simulink model "IEEE9_case"  (R2024b)
settings: Solver=FixedStepAuto  StartTime=0  StopTime=5  FixedStep=1e-7  RelTol=1e-3
values from neighbouring files (symbols this model uses):
  SG_D_1_D = 0.01056    [IEEE9_case_parameters.m]    (also in case1_parameters.m; case2_parameters.m; case3_parameters.m; case4_parameters.m)
  SG_D_1_EnableSaturation = 0    [IEEE9_case_parameters.m]    (also in case1_parameters.m; case2_parameters.m; case3_parameters.m; case4_parameters.m)
  SG_D_1_f0 = 60    [IEEE9_case_parameters.m]    (also in case1_parameters.m; case2_parameters.m; case3_parameters.m; case4_parameters.m)
  SG_D_1_H = 7.5    [IEEE9_case_parameters.m]    (also in case1_parameters.m; case2_parameters.m; case3_parameters.m; case4_parameters.m)
  SG_D_1_K_A = 20    [IEEE9_case_parameters.m]    (also in case1_parameters.m; case2_parameters.m; case3_parameters.m; case4_parameters.m)
  SG_D_1_K_E = 1.000000e+1    (= 10)    [IEEE9_case_parameters.m]    (also in case1_parameters.m; case2_parameters.m; case3_parameters.m; case4_parameters.m)
  SG_D_1_K_F = 2.363    [IEEE9_case_parameters.m]    (also in case1_parameters.m; case2_parameters.m; case3_parameters.m; case4_parameters.m)
  SG_D_1_K_s = 0.5    [IEEE9_case_parameters.m]    (also in case1_parameters.m = 5; case2_parameters.m = 5; case3_parameters.m = 5; case4_parameters.m = 5)
  SG_D_1_R_a = 0.001088    [IEEE9_case_parameters.m]    (also in case1_parameters.m; case2_parameters.m; case3_parameters.m; case4_parameters.m)
  SG_D_1_S_A = 1    [IEEE9_case_parameters.m]    (also in case1_parameters.m; case2_parameters.m; case3_parameters.m; case4_parameters.m)
  SG_D_1_S_B = 0.103    [IEEE9_case_parameters.m]    (also in case1_parameters.m; case2_parameters.m; case3_parameters.m; case4_parameters.m)
  SG_D_1_S_N = 10.659857    [IEEE9_case_parameters.m]    (also in case1_parameters.m; case2_parameters.m; case3_parameters.m; case4_parameters.m)
  SG_D_1_SpeedPara = 200    [IEEE9_case_parameters.m]    (also in case1_parameters.m; case2_parameters.m; case3_parameters.m; case4_parameters.m)
  SG_D_1_T_0 = 0.720173    [IEEE9_case_parameters.m]    (also in case1_parameters.m = 0.755522; case2_parameters.m = 0.808931; case3_parameters.m = 0.869402; case4_parameters.m = 0.729316)
  SG_D_1_T_1 = 0.3    [IEEE9_case_parameters.m]    (also in case1_parameters.m; case2_parameters.m; case3_parameters.m; case4_parameters.m)
  SG_D_1_T_2 = 0.05    [IEEE9_case_parameters.m]    (also in case1_parameters.m; case2_parameters.m; case3_parameters.m; case4_parameters.m)
  SG_D_1_T_3 = 0.02    [IEEE9_case_parameters.m]    (also in case1_parameters.m; case2_parameters.m; case3_parameters.m; case4_parameters.m)
  SG_D_1_T_4 = 0.005    [IEEE9_case_parameters.m]    (also in case1_parameters.m; case2_parameters.m; case3_parameters.m; case4_parameters.m)
  SG_D_1_T_A = 0.02    [IEEE9_case_parameters.m]    (also in case1_parameters.m; case2_parameters.m; case3_parameters.m; case4_parameters.m)
  SG_D_1_T_dd = 8.000000e+0    (= 8)    [IEEE9_case_parameters.m]    (also in case1_parameters.m; case2_parameters.m; case3_parameters.m; case4_parameters.m)
  SG_D_1_T_ddd = 0.04    [IEEE9_case_parameters.m]    (also in case1_parameters.m; case2_parameters.m; case3_parameters.m; case4_parameters.m)
  SG_D_1_T_E = 0.314    [IEEE9_case_parameters.m]    (also in case1_parameters.m; case2_parameters.m; case3_parameters.m; case4_parameters.m)
  SG_D_1_T_F = 0.35    [IEEE9_case_parameters.m]    (also in case1_parameters.m; case2_parameters.m; case3_parameters.m; case4_parameters.m)
  SG_D_1_T_qd = 0.8    [IEEE9_case_parameters.m]    (also in case1_parameters.m; case2_parameters.m; case3_parameters.m; case4_parameters.m)
  SG_D_1_T_qdd = 0.02    [IEEE9_case_parameters.m]    (also in case1_parameters.m; case2_parameters.m; case3_parameters.m; case4_parameters.m)
  SG_D_1_T_speed = 0.1    [IEEE9_case_parameters.m]    (also in case1_parameters.m = 200; case2_parameters.m = 200; case3_parameters.m = 200; case4_parameters.m = 200)
  SG_D_1_T_w = 0.5    [IEEE9_case_parameters.m]    (also in case1_parameters.m; case2_parameters.m; case3_parameters.m; case4_parameters.m)
  SG_D_1_V_ref = 1.990276    [IEEE9_case_parameters.m]    (also in case1_parameters.m = 2.042296; case2_parameters.m = 2.051388; case3_parameters.m = 2.089584; case4_parameters.m = 2.01845)
  SG_D_1_w_ref = 376.991118    [IEEE9_case_parameters.m]    (also in case1_parameters.m; case2_parameters.m; case3_parameters.m; case4_parameters.m)
  SG_D_1_wb = 6.000000e+1    (= 60)    [IEEE9_case_parameters.m]    (also in case1_parameters.m; case2_parameters.m; case3_parameters.m; case4_parameters.m)
  SG_D_1_x_d = 1.9    [IEEE9_case_parameters.m]    (also in case1_parameters.m; case2_parameters.m; case3_parameters.m; case4_parameters.m)
  SG_D_1_x_dd = 0.302    [IEEE9_case_parameters.m]    (also in case1_parameters.m; case2_parameters.m; case3_parameters.m; case4_parameters.m)
  SG_D_1_x_ddd = 0.204    [IEEE9_case_parameters.m]    (also in case1_parameters.m; case2_parameters.m; case3_parameters.m; case4_parameters.m)
  SG_D_1_x_l = 0.05    [IEEE9_case_parameters.m]    (also in case1_parameters.m; case2_parameters.m; case3_parameters.m; case4_parameters.m)
  SG_D_1_x_q = 1.3    [IEEE9_case_parameters.m]    (also in case1_parameters.m; case2_parameters.m; case3_parameters.m; case4_parameters.m)
  SG_D_1_x_qd = 0.5    [IEEE9_case_parameters.m]    (also in case1_parameters.m; case2_parameters.m; case3_parameters.m; case4_parameters.m)
  SG_D_1_x_qdd = 0.3    [IEEE9_case_parameters.m]    (also in case1_parameters.m; case2_parameters.m; case3_parameters.m; case4_parameters.m)
  SG_D_2_D = 0.02    [IEEE9_case_parameters.m]    (also in case1_parameters.m; case2_parameters.m; case3_parameters.m; case4_parameters.m)
  SG_D_2_EnableSaturation = 0    [IEEE9_case_parameters.m]    (also in case1_parameters.m; case2_parameters.m; case3_parameters.m; case4_parameters.m)
  SG_D_2_f0 = 60    [IEEE9_case_parameters.m]    (also in case1_parameters.m; case2_parameters.m; case3_parameters.m; case4_parameters.m)
  SG_D_2_H = 8.000000e+0    (= 8)    [IEEE9_case_parameters.m]    (also in case1_parameters.m; case2_parameters.m; case3_parameters.m; case4_parameters.m)
  SG_D_2_K_A = 20    [IEEE9_case_parameters.m]    (also in case1_parameters.m; case2_parameters.m; case3_parameters.m; case4_parameters.m)
  SG_D_2_K_E = 1.000000e+1    (= 10)    [IEEE9_case_parameters.m]    (also in case1_parameters.m; case2_parameters.m; case3_parameters.m; case4_parameters.m)
  SG_D_2_K_F = 2.363    [IEEE9_case_parameters.m]    (also in case1_parameters.m; case2_parameters.m; case3_parameters.m; case4_parameters.m)
  SG_D_2_K_s = 0.5    [IEEE9_case_parameters.m]    (also in case1_parameters.m = 4; case2_parameters.m = 4; case3_parameters.m = 4; case4_parameters.m = 4)
  SG_D_2_R_a = 0.001088    [IEEE9_case_parameters.m]    (also in case1_parameters.m; case2_parameters.m; case3_parameters.m; case4_parameters.m)
  SG_D_2_S_A = 1    [IEEE9_case_parameters.m]    (also in case1_parameters.m; case2_parameters.m; case3_parameters.m; case4_parameters.m)
  SG_D_2_S_B = 0.103    [IEEE9_case_parameters.m]    (also in case1_parameters.m; case2_parameters.m; case3_parameters.m; case4_parameters.m)
  SG_D_2_S_N = 10.659857    [IEEE9_case_parameters.m]    (also in case1_parameters.m; case2_parameters.m; case3_parameters.m; case4_parameters.m)
  SG_D_2_SpeedPara = 200    [IEEE9_case_parameters.m]    (also in case1_parameters.m; case2_parameters.m; case3_parameters.m; case4_parameters.m)
  SG_D_2_T_0 = 1.632913    [IEEE9_case_parameters.m]    (also in case1_parameters.m = 1.632925; case2_parameters.m = 1.632915; case3_parameters.m = 1.632914; case4_parameters.m = 1.632927)
  SG_D_2_T_1 = 0.2    [IEEE9_case_parameters.m]    (also in case1_parameters.m; case2_parameters.m; case3_parameters.m; case4_parameters.m)
  SG_D_2_T_2 = 0.05    [IEEE9_case_parameters.m]    (also in case1_parameters.m; case2_parameters.m; case3_parameters.m; case4_parameters.m)
  SG_D_2_T_3 = 0.02    [IEEE9_case_parameters.m]    (also in case1_parameters.m; case2_parameters.m; case3_parameters.m; case4_parameters.m)
  SG_D_2_T_4 = 0.005    [IEEE9_case_parameters.m]    (also in case1_parameters.m; case2_parameters.m; case3_parameters.m; case4_parameters.m)
  SG_D_2_T_A = 0.02    [IEEE9_case_parameters.m]    (also in case1_parameters.m; case2_parameters.m; case3_parameters.m; case4_parameters.m)
  SG_D_2_T_dd = 7.9    [IEEE9_case_parameters.m]    (also in case1_parameters.m; case2_parameters.m; case3_parameters.m; case4_parameters.m)
  SG_D_2_T_ddd = 0.04    [IEEE9_case_parameters.m]    (also in case1_parameters.m; case2_parameters.m; case3_parameters.m; case4_parameters.m)
  SG_D_2_T_E = 0.314    [IEEE9_case_parameters.m]    (also in case1_parameters.m; case2_parameters.m; case3_parameters.m; case4_parameters.m)
  SG_D_2_T_F = 0.35    [IEEE9_case_parameters.m]    (also in case1_parameters.m; case2_parameters.m; case3_parameters.m; case4_parameters.m)
  SG_D_2_T_qd = 0.8    [IEEE9_case_parameters.m]    (also in case1_parameters.m; case2_parameters.m; case3_parameters.m; case4_parameters.m)
  SG_D_2_T_qdd = 0.015    [IEEE9_case_parameters.m]    (also in case1_parameters.m; case2_parameters.m; case3_parameters.m; case4_parameters.m)
  SG_D_2_T_speed = 0.1    [IEEE9_case_parameters.m]    (also in case1_parameters.m = 150; case2_parameters.m = 150; case3_parameters.m = 150; case4_parameters.m = 150)
  SG_D_2_T_w = 0.35    [IEEE9_case_parameters.m]    (also in case1_parameters.m; case2_parameters.m; case3_parameters.m; case4_parameters.m)
  SG_D_2_V_ref = 2.58547    [IEEE9_case_parameters.m]    (also in case1_parameters.m = 2.597896; case2_parameters.m = 2.587136; case3_parameters.m = 2.586042; case4_parameters.m = 2.599679)
  SG_D_2_w_ref = 376.991118    [IEEE9_case_parameters.m]    (also in case1_parameters.m; case2_parameters.m; case3_parameters.m; case4_parameters.m)
  SG_D_2_wb = 6.000000e+1    (= 60)    [IEEE9_case_parameters.m]    (also in case1_parameters.m; case2_parameters.m; case3_parameters.m; case4_parameters.m)
  SG_D_2_x_d = 1.8    [IEEE9_case_parameters.m]    (also in case1_parameters.m; case2_parameters.m; case3_parameters.m; case4_parameters.m)
  SG_D_2_x_dd = 0.302    [IEEE9_case_parameters.m]    (also in case1_parameters.m; case2_parameters.m; case3_parameters.m; case4_parameters.m)
  SG_D_2_x_ddd = 0.204    [IEEE9_case_parameters.m]    (also in case1_parameters.m; case2_parameters.m; case3_parameters.m; case4_parameters.m)
  SG_D_2_x_l = 0.05    [IEEE9_case_parameters.m]    (also in case1_parameters.m; case2_parameters.m; case3_parameters.m; case4_parameters.m)
  SG_D_2_x_q = 1.25    [IEEE9_case_parameters.m]    (also in case1_parameters.m; case2_parameters.m; case3_parameters.m; case4_parameters.m)
  SG_D_2_x_qd = 0.5    [IEEE9_case_parameters.m]    (also in case1_parameters.m; case2_parameters.m; case3_parameters.m; case4_parameters.m)
  SG_D_2_x_qdd = 0.3    [IEEE9_case_parameters.m]    (also in case1_parameters.m; case2_parameters.m; case3_parameters.m; case4_parameters.m)
  SG_D_3_D = 0.02    [IEEE9_case_parameters.m]    (also in case1_parameters.m; case2_parameters.m; case3_parameters.m; case4_parameters.m)
  SG_D_3_EnableSaturation = 0    [IEEE9_case_parameters.m]    (also in case1_parameters.m; case2_parameters.m; case3_parameters.m; case4_parameters.m)
  SG_D_3_f0 = 60    [IEEE9_case_parameters.m]    (also in case1_parameters.m; case2_parameters.m; case3_parameters.m; case4_parameters.m)
  SG_D_3_H = 7.7    [IEEE9_case_parameters.m]    (also in case1_parameters.m; case2_parameters.m; case3_parameters.m; case4_parameters.m)
  SG_D_3_K_A = 20    [IEEE9_case_parameters.m]    (also in case1_parameters.m; case2_parameters.m; case3_parameters.m; case4_parameters.m)
  SG_D_3_K_E = 1.000000e+1    (= 10)    [IEEE9_case_parameters.m]    (also in case1_parameters.m; case2_parameters.m; case3_parameters.m; case4_parameters.m)
  SG_D_3_K_F = 2.363    [IEEE9_case_parameters.m]    (also in case1_parameters.m; case2_parameters.m; case3_parameters.m; case4_parameters.m)
  SG_D_3_K_s = 0.2    [IEEE9_case_parameters.m]    (also in case1_parameters.m = 2; case2_parameters.m = 2; case3_parameters.m = 2; case4_parameters.m = 2)
  SG_D_3_R_a = 0.001088    [IEEE9_case_parameters.m]    (also in case1_parameters.m; case2_parameters.m; case3_parameters.m; case4_parameters.m)
  SG_D_3_S_A = 1    [IEEE9_case_parameters.m]    (also in case1_parameters.m; case2_parameters.m; case3_parameters.m; case4_parameters.m)
  SG_D_3_S_B = 0.103    [IEEE9_case_parameters.m]    (also in case1_parameters.m; case2_parameters.m; case3_parameters.m; case4_parameters.m)
  SG_D_3_S_N = 10.659857    [IEEE9_case_parameters.m]    (also in case1_parameters.m; case2_parameters.m; case3_parameters.m; case4_parameters.m)
  SG_D_3_SpeedPara = 200    [IEEE9_case_parameters.m]    (also in case1_parameters.m; case2_parameters.m; case3_parameters.m; case4_parameters.m)
  SG_D_3_T_0 = 0.850788    [IEEE9_case_parameters.m]    (also in case1_parameters.m = 0.850786; case2_parameters.m = 0.850787; case3_parameters.m; case4_parameters.m = 0.850786)
  SG_D_3_T_1 = 0.2    [IEEE9_case_parameters.m]    (also in case1_parameters.m; case2_parameters.m; case3_parameters.m; case4_parameters.m)
  SG_D_3_T_2 = 0.05    [IEEE9_case_parameters.m]    (also in case1_parameters.m; case2_parameters.m; case3_parameters.m; case4_parameters.m)
  SG_D_3_T_3 = 0.02    [IEEE9_case_parameters.m]    (also in case1_parameters.m; case2_parameters.m; case3_parameters.m; case4_parameters.m)
  SG_D_3_T_4 = 0.005    [IEEE9_case_parameters.m]    (also in case1_parameters.m; case2_parameters.m; case3_parameters.m; case4_parameters.m)
  SG_D_3_T_A = 0.02    [IEEE9_case_parameters.m]    (also in case1_parameters.m; case2_parameters.m; case3_parameters.m; case4_parameters.m)
  SG_D_3_T_dd = 8.1    [IEEE9_case_parameters.m]    (also in case1_parameters.m; case2_parameters.m; case3_parameters.m; case4_parameters.m)
  SG_D_3_T_ddd = 0.04    [IEEE9_case_parameters.m]    (also in case1_parameters.m; case2_parameters.m; case3_parameters.m; case4_parameters.m)
  SG_D_3_T_E = 0.314    [IEEE9_case_parameters.m]    (also in case1_parameters.m; case2_parameters.m; case3_parameters.m; case4_parameters.m)
  SG_D_3_T_F = 0.35    [IEEE9_case_parameters.m]    (also in case1_parameters.m; case2_parameters.m; case3_parameters.m; case4_parameters.m)
  SG_D_3_T_qd = 0.8    [IEEE9_case_parameters.m]    (also in case1_parameters.m; case2_parameters.m; case3_parameters.m; case4_parameters.m)
  SG_D_3_T_qdd = 0.015    [IEEE9_case_parameters.m]    (also in case1_parameters.m; case2_parameters.m; case3_parameters.m; case4_parameters.m)
  SG_D_3_T_speed = 0.1    [IEEE9_case_parameters.m]    (also in case1_parameters.m = 180; case2_parameters.m = 180; case3_parameters.m = 180; case4_parameters.m = 180)
  SG_D_3_T_w = 0.4    [IEEE9_case_parameters.m]    (also in case1_parameters.m; case2_parameters.m; case3_parameters.m; case4_parameters.m)
  SG_D_3_V_ref = 1.892727    [IEEE9_case_parameters.m]    (also in case1_parameters.m = 1.906439; case2_parameters.m = 1.895535; case3_parameters.m = 1.892105; case4_parameters.m = 1.906598)
  SG_D_3_w_ref = 376.991118    [IEEE9_case_parameters.m]    (also in case1_parameters.m; case2_parameters.m; case3_parameters.m; case4_parameters.m)
  SG_D_3_wb = 6.000000e+1    (= 60)    [IEEE9_case_parameters.m]    (also in case1_parameters.m; case2_parameters.m; case3_parameters.m; case4_parameters.m)
  SG_D_3_x_d = 1.85    [IEEE9_case_parameters.m]    (also in case1_parameters.m; case2_parameters.m; case3_parameters.m; case4_parameters.m)
  SG_D_3_x_dd = 0.302    [IEEE9_case_parameters.m]    (also in case1_parameters.m; case2_parameters.m; case3_parameters.m; case4_parameters.m)
  SG_D_3_x_ddd = 0.204    [IEEE9_case_parameters.m]    (also in case1_parameters.m; case2_parameters.m; case3_parameters.m; case4_parameters.m)
  SG_D_3_x_l = 0.05    [IEEE9_case_parameters.m]    (also in case1_parameters.m; case2_parameters.m; case3_parameters.m; case4_parameters.m)
  SG_D_3_x_q = 1.2    [IEEE9_case_parameters.m]    (also in case1_parameters.m; case2_parameters.m; case3_parameters.m; case4_parameters.m)
  SG_D_3_x_qd = 0.5    [IEEE9_case_parameters.m]    (also in case1_parameters.m; case2_parameters.m; case3_parameters.m; case4_parameters.m)
  SG_D_3_x_qdd = 0.3    [IEEE9_case_parameters.m]    (also in case1_parameters.m; case2_parameters.m; case3_parameters.m; case4_parameters.m)
(part 1 of 12)
settings Model: SimulationMode=accelerator  Creator=Greg  LastModifiedBy=Greg
settings DataIOCC: ReturnWorkspaceOutputs=off

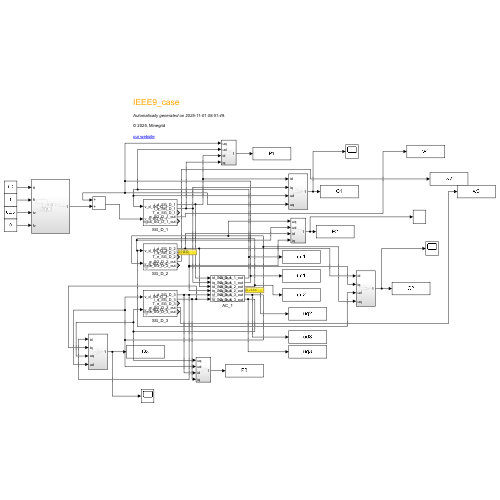
[thumbnail: Simulink's stored preview of the top-level diagram]
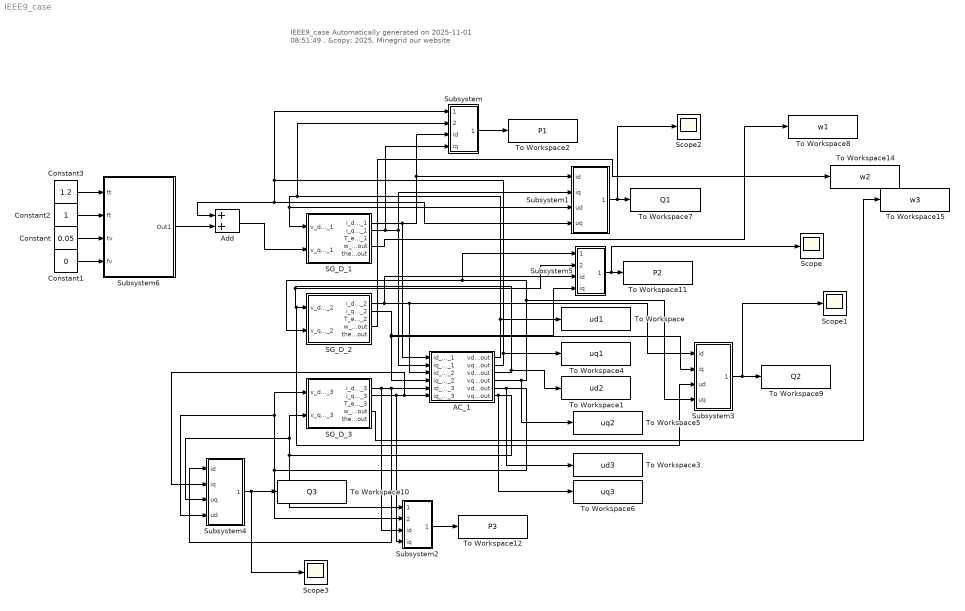
== system IEEE9_case ==
  note: IEEE9_case
      | Automatically generated on 2025-11-01 08:51:49 .
      | &copy; 2025, Minegrid
      | our website
  AC_1 : Subsystem  mask(AC_1){}
      mask help: Parameters Interface of AC_1
  Add : Sum
  Constant : Constant  Value=0.05
  Constant1 : Constant  Value=0
  Constant2 : Constant
  Constant3 : Constant  Value=1.2
  SG_D_1 : Subsystem  mask(SG_D_1){T_0=SG_D_1_T_0, w_ref=SG_D_1_w_ref, V_ref=SG_D_1_V_ref, x_d=SG_D_1_x_d, x_dd=SG_D_1_x_dd, x_ddd=SG_D_1_x_ddd, x_q=SG_D_1_x_q, x_qd=SG_D_1_x_qd, x_qdd=SG_D_1_x_qdd, x_l=SG_D_1_x_l, R_a=SG_D_1_R_a, T_dd=SG_D_1_T_dd, T_ddd=SG_D_1_T_ddd, T_qd=SG_D_1_T_qd, T_qdd=SG_D_1_T_qdd, H=SG_D_1_H, D=SG_D_1_D, SpeedPara=SG_D_1_SpeedPara, K_A=SG_D_1_K_A, EnableSaturation=SG_D_1_EnableSaturation, f0=SG_D_1_f0, T_speed=SG_D_1_T_speed, T_E=SG_D_1_T_E, T_A=SG_D_1_T_A, T_F=SG_D_1_T_F, K_E=SG_D_1_K_E, K_F=SG_D_1_K_F, K_s=SG_D_1_K_s, T_1=SG_D_1_T_1, T_2=SG_D_1_T_2, T_3=SG_D_1_T_3, T_4=SG_D_1_T_4, T_w=SG_D_1_T_w, wb=SG_D_1_wb, S_A=SG_D_1_S_A, S_B=SG_D_1_S_B, S_N=SG_D_1_S_N}
      mask help: Parameters Interface of SG_D_1
  SG_D_2 : Subsystem  mask(SG_D_2){T_0=SG_D_2_T_0, w_ref=SG_D_2_w_ref, V_ref=SG_D_2_V_ref, x_d=SG_D_2_x_d, x_dd=SG_D_2_x_dd, x_ddd=SG_D_2_x_ddd, x_q=SG_D_2_x_q, x_qd=SG_D_2_x_qd, x_qdd=SG_D_2_x_qdd, x_l=SG_D_2_x_l, R_a=SG_D_2_R_a, T_dd=SG_D_2_T_dd, T_ddd=SG_D_2_T_ddd, T_qd=SG_D_2_T_qd, T_qdd=SG_D_2_T_qdd, H=SG_D_2_H, D=SG_D_2_D, SpeedPara=SG_D_2_SpeedPara, K_A=SG_D_2_K_A, EnableSaturation=SG_D_2_EnableSaturation, f0=SG_D_2_f0, T_speed=SG_D_2_T_speed, T_E=SG_D_2_T_E, T_A=SG_D_2_T_A, T_F=SG_D_2_T_F, K_E=SG_D_2_K_E, K_F=SG_D_2_K_F, K_s=SG_D_2_K_s, T_1=SG_D_2_T_1, T_2=SG_D_2_T_2, T_3=SG_D_2_T_3, T_4=SG_D_2_T_4, T_w=SG_D_2_T_w, wb=SG_D_2_wb, S_A=SG_D_2_S_A, S_B=SG_D_2_S_B, S_N=SG_D_2_S_N}
      mask help: Parameters Interface of SG_D_2
  SG_D_3 : Subsystem  mask(SG_D_3){T_0=SG_D_3_T_0, w_ref=SG_D_3_w_ref, V_ref=SG_D_3_V_ref, x_d=SG_D_3_x_d, x_dd=SG_D_3_x_dd, x_ddd=SG_D_3_x_ddd, x_q=SG_D_3_x_q, x_qd=SG_D_3_x_qd, x_qdd=SG_D_3_x_qdd, x_l=SG_D_3_x_l, R_a=SG_D_3_R_a, T_dd=SG_D_3_T_dd, T_ddd=SG_D_3_T_ddd, T_qd=SG_D_3_T_qd, T_qdd=SG_D_3_T_qdd, H=SG_D_3_H, D=SG_D_3_D, SpeedPara=SG_D_3_SpeedPara, K_A=SG_D_3_K_A, EnableSaturation=SG_D_3_EnableSaturation, f0=SG_D_3_f0, T_speed=SG_D_3_T_speed, T_E=SG_D_3_T_E, T_A=SG_D_3_T_A, T_F=SG_D_3_T_F, K_E=SG_D_3_K_E, K_F=SG_D_3_K_F, K_s=SG_D_3_K_s, T_1=SG_D_3_T_1, T_2=SG_D_3_T_2, T_3=SG_D_3_T_3, T_4=SG_D_3_T_4, T_w=SG_D_3_T_w, wb=SG_D_3_wb, S_A=SG_D_3_S_A, S_B=SG_D_3_S_B, S_N=SG_D_3_S_N}
      mask help: Parameters Interface of SG_D_3
  Scope{,1..3} (4 alike) : Scope
  Subsystem : Subsystem
  Subsystem1 : Subsystem
  Subsystem2 : Subsystem
  Subsystem3 : Subsystem
  Subsystem4 : Subsystem
  Subsystem5 : Subsystem
  Subsystem6 : Subsystem
  To Workspace : ToWorkspace  VariableName=ud1  SampleTime=-1
  To Workspace1 : ToWorkspace  VariableName=ud2  SampleTime=-1
  To Workspace10 : ToWorkspace  VariableName=Q3  SampleTime=-1
  To Workspace11 : ToWorkspace  VariableName=P2  SampleTime=-1
  To Workspace12 : ToWorkspace  VariableName=P3  SampleTime=-1
  To Workspace14 : ToWorkspace  VariableName=w2  SampleTime=-1
  To Workspace15 : ToWorkspace  VariableName=w3  SampleTime=-1
  To Workspace2 : ToWorkspace  VariableName=P1  SampleTime=-1
  To Workspace3 : ToWorkspace  VariableName=ud3  SampleTime=-1
  To Workspace4 : ToWorkspace  VariableName=uq1  SampleTime=-1
  To Workspace5 : ToWorkspace  VariableName=uq2  SampleTime=-1
  To Workspace6 : ToWorkspace  VariableName=uq3  SampleTime=-1
  To Workspace7 : ToWorkspace  VariableName=Q1  SampleTime=-1
  To Workspace8 : ToWorkspace  VariableName=w1  SampleTime=-1
  To Workspace9 : ToWorkspace  VariableName=Q2  SampleTime=-1
  wires:
  SG_D_1/1(i_d_SG_D_1) -> Subsystem1/1(id), Subsystem/3(id), AC_1/1(id_SG_D_1)
  SG_D_2/1(i_d_SG_D_2) -> Subsystem5/3(id), AC_1/3(id_SG_D_2), Subsystem3/1(id)
  SG_D_3/1(i_d_SG_D_3) -> Subsystem2/3(id), Subsystem4/1(id), AC_1/5(id_SG_D_3)
  AC_1/2(vq_bus_1_out) -> To Workspace4/1, Subsystem/1(uq), Add/1, Subsystem1/4(uq)
  SG_D_3/2(i_q_SG_D_3) -> Subsystem2/4(iq), Subsystem4/2(iq), AC_1/6(iq_SG_D_3)
  AC_1/3(vd_bus_2_out) -> To Workspace1/1, Subsystem3/3(ud), SG_D_2/1(v_d_SG_D_2), Subsystem5/2(ud)
  AC_1/4(vq_bus_2_out) -> To Workspace5/1, SG_D_2/2(v_q_SG_D_2), Subsystem5/1(uq), Subsystem3/4(uq)
  AC_1/5(vd_bus_3_out) -> To Workspace3/1, SG_D_3/1(v_d_SG_D_3), Subsystem4/4(ud), Subsystem2/2(ud)
  AC_1/6(vq_bus_3_out) -> To Workspace6/1, SG_D_3/2(v_q_SG_D_3), Subsystem4/3(uq), Subsystem2/1(uq)
  AC_1/1(vd_bus_1_out) -> To Workspace/1, Subsystem/2(ud), Subsystem1/3(ud), SG_D_1/1(v_d_SG_D_1)
  SG_D_1/2(i_q_SG_D_1) -> Subsystem/4(iq), AC_1/2(iq_SG_D_1), Subsystem1/2(iq)
  Subsystem/1(Out1) -> To Workspace2/1
  Subsystem1/1(Out1) -> Scope2/1, To Workspace7/1
  Subsystem5/1(Out1) -> Scope/1, To Workspace11/1
  Subsystem2/1(Out1) -> To Workspace12/1
  SG_D_2/2(i_q_SG_D_2) -> AC_1/4(iq_SG_D_2), Subsystem3/2(iq), Subsystem5/4(iq)
  Subsystem3/1(Out1) -> Scope1/1, To Workspace9/1
  Subsystem4/1(Out1) -> Scope3/1, To Workspace10/1
  SG_D_1/4(w_SG_D_1_out) -> To Workspace8/1
  SG_D_2/4(w_SG_D_2_out) -> To Workspace14/1
  SG_D_3/4(w_SG_D_3_out) -> To Workspace15/1
  Constant1/1 -> Subsystem6/4(fv)
  Constant2/1 -> Subsystem6/2(ft)
  Constant3/1 -> Subsystem6/1(tt)
  Constant/1 -> Subsystem6/3(tv)
  Subsystem6/1(Out1) -> Add/2
  Add/1 -> SG_D_1/2(v_q_SG_D_1)

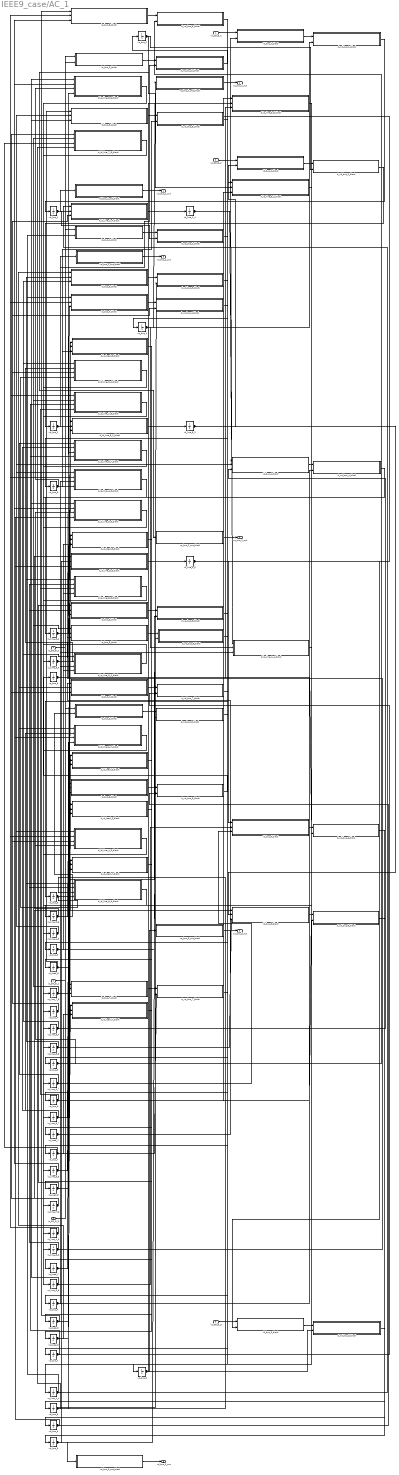
== system IEEE9_case/AC_1 ==
  id_SG_D_1 : Inport
  iq_SG_D_1 : Inport  Port=2
  id_SG_D_2 : Inport  Port=3
  iq_SG_D_2 : Inport  Port=4
  id_SG_D_3 : Inport  Port=5
  iq_SG_D_3 : Inport  Port=6
  d_id_line_1_4_block : Subsystem
  d_id_line_3_6_block : Subsystem
  d_id_line_4_5_block : Subsystem
  d_id_line_5_6_block : Subsystem
  d_id_line_6_7_block : Subsystem
  d_id_line_7_8_block : Subsystem
  d_id_line_8_2_block : Subsystem
  d_id_line_8_9_block : Subsystem
  d_id_line_9_4_block : Subsystem
  d_id_load_5_block : Subsystem
  d_id_load_7_block : Subsystem
  d_id_load_9_block : Subsystem
  d_iq_line_1_4_block : Subsystem
  d_iq_line_3_6_block : Subsystem
  d_iq_line_4_5_block : Subsystem
  d_iq_line_5_6_block : Subsystem
  d_iq_line_6_7_block : Subsystem
  d_iq_line_7_8_block : Subsystem
  d_iq_line_8_2_block : Subsystem
  d_iq_line_8_9_block : Subsystem
  d_iq_line_9_4_block : Subsystem
  d_iq_load_5_block : Subsystem
  d_iq_load_7_block : Subsystem
  d_iq_load_9_block : Subsystem
  d_vd_bus_1_block : Subsystem
  d_vd_bus_2_block : Subsystem
  d_vd_bus_3_block : Subsystem
  d_vd_bus_4_block : Subsystem
  d_vd_bus_5_block : Subsystem
  d_vd_bus_6_block : Subsystem
  d_vd_bus_7_block : Subsystem
  d_vd_bus_8_block : Subsystem
  d_vd_bus_9_block : Subsystem
  d_vq_bus_1_block : Subsystem
  d_vq_bus_2_block : Subsystem
  d_vq_bus_3_block : Subsystem
  d_vq_bus_4_block : Subsystem
  d_vq_bus_5_block : Subsystem
  d_vq_bus_6_block : Subsystem
  d_vq_bus_7_block : Subsystem
  d_vq_bus_8_block : Subsystem
  d_vq_bus_9_block : Subsystem
  id_bus_1_block : Subsystem
  id_bus_2_block : Subsystem
  id_bus_3_block : Subsystem
  id_bus_4_block : Subsystem
  id_bus_5_block : Subsystem
  id_bus_6_block : Subsystem
  id_bus_7_block : Subsystem
  id_bus_8_block : Subsystem
  id_bus_9_block : Subsystem
  id_line_1_4 : Integrator  InitialCondition=0.7195
  id_line_3_6 : Integrator  InitialCondition=0.844
  id_line_4_5 : Integrator  InitialCondition=0.308
  id_line_5_6 : Integrator  InitialCondition=-0.6084
  id_line_6_7 : Integrator  InitialCondition=0.2452
  id_line_7_8 : Integrator  InitialCondition=-0.7713
  id_line_8_2 : Integrator  InitialCondition=-1.6311
  id_line_8_9 : Integrator  InitialCondition=0.8749
  id_line_9_4 : Integrator  InitialCondition=-0.4046
  id_load_5 : Integrator  InitialCondition=0.898817607082261
  id_load_7 : Integrator  InitialCondition=1.0183565162188208
  id_load_9 : Integrator  InitialCondition=1.2619557605717109
  iq_bus_1_block : Subsystem
  iq_bus_2_block : Subsystem
  iq_bus_3_block : Subsystem
  iq_bus_4_block : Subsystem
  iq_bus_5_block : Subsystem
  iq_bus_6_block : Subsystem
  iq_bus_7_block : Subsystem
  iq_bus_8_block : Subsystem
  iq_bus_9_block : Subsystem
  iq_line_1_4 : Integrator  InitialCondition=-0.2407
  iq_line_3_6 : Integrator  InitialCondition=0.1071
  iq_line_4_5 : Integrator  InitialCondition=-0.085
  iq_line_5_6 : Integrator  InitialCondition=0.0353
  iq_line_6_7 : Integrator  InitialCondition=-0.1419
  iq_line_7_8 : Integrator  InitialCondition=0.0257
  iq_line_8_2 : Integrator  InitialCondition=-0.1312
  iq_line_8_9 : Integrator  InitialCondition=-0.0692
  iq_line_9_4 : Integrator  InitialCondition=0.3203
  iq_load_5 : Integrator  InitialCondition=-0.37142447893959263
  iq_load_7 : Integrator  InitialCondition=-0.34407079769452764
  iq_load_9 : Integrator  InitialCondition=-0.6196286093512099
  vd_bus_1 : Integrator  InitialCondition=1.0
  vd_bus_1_out_block : Subsystem
  vd_bus_2 : Integrator  InitialCondition=0.9857952451733694
  vd_bus_2_out_block : Subsystem
  vd_bus_3 : Integrator  InitialCondition=0.9965349784480291
  vd_bus_3_out_block : Subsystem
  vd_bus_4 : Integrator  InitialCondition=0.9861362779327475
  vd_bus_5 : Integrator  InitialCondition=0.9730754311923555
  vd_bus_6 : Integrator  InitialCondition=1.0028088352065478
  vd_bus_7 : Integrator  InitialCondition=0.9855868856760395
  vd_bus_8 : Integrator  InitialCondition=0.9939961188157862
  vd_bus_9 : Integrator  InitialCondition=0.9548625268660215
  vq_bus_1 : Integrator  InitialCondition=0.0
  vq_bus_1_out_block : Subsystem
  vq_bus_2 : Integrator  InitialCondition=0.16795158407581826
  vq_bus_2_out_block : Subsystem
  vq_bus_3 : Integrator  InitialCondition=0.08317473612573835
  vq_bus_3_out_block : Subsystem
  vq_bus_4 : Integrator  InitialCondition=-0.04144590802322367
  vq_bus_5 : Integrator  InitialCondition=-0.06833870911689703
  vq_bus_6 : Integrator  InitialCondition=0.03371518392178962
  vq_bus_7 : Integrator  InitialCondition=0.01069206498389038
  vq_bus_8 : Integrator  InitialCondition=0.06600581865802534
  vq_bus_9 : Integrator  InitialCondition=-0.07263340166698863
  vd_bus_1_out : Outport
  vq_bus_1_out : Outport  Port=2
  vd_bus_2_out : Outport  Port=3
  vq_bus_2_out : Outport  Port=4
  vd_bus_3_out : Outport  Port=5
  vq_bus_3_out : Outport  Port=6
  wires:
  id_line_8_2/1 -> id_bus_2_block/2(State_id_line_8_2_3c453), id_bus_8_block/2(State_id_line_8_2_3341e), d_iq_line_8_2_block/1(State_id_line_8_2_6fbbf)
  d_id_line_9_4_block/1(Blockout_d_id_line_9_4_80f4f) -> id_line_9_4/1
  vq_bus_5/1 -> d_iq_load_5_block/3(State_vq_bus_5_98bbe), d_iq_line_4_5_block/4(State_vq_bus_5_00127), d_iq_line_5_6_block/3(State_vq_bus_5_5d45c), d_vd_bus_5_block/2(State_vq_bus_5_adcb7)
  iq_line_8_2/1 -> d_id_line_8_2_block/1(State_iq_line_8_2_9277c), iq_bus_2_block/2(State_iq_line_8_2_dbe3b), iq_bus_8_block/2(State_iq_line_8_2_b7626)
  iq_bus_1_block/1(Blockout_iq_bus_1_a22e6) -> d_vq_bus_1_block/1(Alge_iq_bus_1_fd912)
  id_line_7_8/1 -> d_id_line_7_8_block/1(State_id_line_7_8_54820), id_bus_7_block/3(State_id_line_7_8_cc267), d_iq_line_7_8_block/1(State_id_line_7_8_c97aa), id_bus_8_block/1(State_id_line_7_8_7df9d)
  d_id_line_3_6_block/1(Blockout_d_id_line_3_6_e83e3) -> id_line_3_6/1
  vq_bus_2/1 -> d_iq_line_8_2_block/2(State_vq_bus_2_442ae), vq_bus_2_out_block/1(State_vq_bus_2_ae5be), d_vd_bus_2_block/2(State_vq_bus_2_66edc)
  id_SG_D_2/1 -> id_bus_2_block/1(Input_id_SG_D_2_61c78)
  id_SG_D_1/1 -> id_bus_1_block/1(Input_id_SG_D_1_af302)
  iq_bus_9_block/1(Blockout_iq_bus_9_298a2) -> d_vq_bus_9_block/1(Alge_iq_bus_9_8c1c8)
  vq_bus_2_out_block/1(Blockout_vq_bus_2_out_a1917) -> vq_bus_2_out/1
  d_id_line_1_4_block/1(Blockout_d_id_line_1_4_47f01) -> id_line_1_4/1
  iq_SG_D_3/1 -> iq_bus_3_block/1(Input_iq_SG_D_3_bb505)
  id_bus_3_block/1(Blockout_id_bus_3_4fcdf) -> d_vd_bus_3_block/1(Alge_id_bus_3_a6e23)
  id_bus_8_block/1(Blockout_id_bus_8_96b63) -> d_vd_bus_8_block/1(Alge_id_bus_8_85559)
  iq_line_5_6/1 -> d_id_line_5_6_block/2(State_iq_line_5_6_e0044), d_iq_line_5_6_block/2(State_iq_line_5_6_c9448), iq_bus_5_block/3(State_iq_line_5_6_863ab), iq_bus_6_block/2(State_iq_line_5_6_aa0cd)
  iq_SG_D_2/1 -> iq_bus_2_block/1(Input_iq_SG_D_2_0132f)
  vd_bus_3_out_block/1(Blockout_vd_bus_3_out_d8755) -> vd_bus_3_out/1
  d_iq_line_8_2_block/1(Blockout_d_iq_line_8_2_35d70) -> iq_line_8_2/1
  d_vd_bus_4_block/1(Blockout_d_vd_bus_4_55aab) -> vd_bus_4/1
  id_SG_D_3/1 -> id_bus_3_block/1(Input_id_SG_D_3_1023f)
  d_id_line_6_7_block/1(Blockout_d_id_line_6_7_12f87) -> id_line_6_7/1
  iq_SG_D_1/1 -> iq_bus_1_block/1(Input_iq_SG_D_1_4742e)
  id_bus_9_block/1(Blockout_id_bus_9_9113d) -> d_vd_bus_9_block/1(Alge_id_bus_9_44435)
  vq_bus_3_out_block/1(Blockout_vq_bus_3_out_d8ffc) -> vq_bus_3_out/1
  iq_bus_8_block/1(Blockout_iq_bus_8_966d9) -> d_vq_bus_8_block/1(Alge_iq_bus_8_0a88b)
  d_id_line_8_2_block/1(Blockout_d_id_line_8_2_95461) -> id_line_8_2/1
  d_vd_bus_1_block/1(Blockout_d_vd_bus_1_137dc) -> vd_bus_1/1
  iq_bus_7_block/1(Blockout_iq_bus_7_2f8a2) -> d_vq_bus_7_block/1(Alge_iq_bus_7_41fff)
  id_bus_7_block/1(Blockout_id_bus_7_6ffd7) -> d_vd_bus_7_block/1(Alge_id_bus_7_08ef0)
  vd_bus_4/1 -> d_vq_bus_4_block/2(State_vd_bus_4_b9421), d_id_line_4_5_block/3(State_vd_bus_4_0a732), d_id_line_9_4_block/3(State_vd_bus_4_38073), d_id_line_1_4_block/3(State_vd_bus_4_87ca3)
  iq_bus_5_block/1(Blockout_iq_bus_5_ca42e) -> d_vq_bus_5_block/1(Alge_iq_bus_5_29d6a)
  d_vq_bus_2_block/1(Blockout_d_vq_bus_2_09653) -> vq_bus_2/1
  d_id_load_7_block/1(Blockout_d_id_load_7_0150f) -> id_load_7/1
  iq_bus_6_block/1(Blockout_iq_bus_6_857b2) -> d_vq_bus_6_block/1(Alge_iq_bus_6_36995)
  iq_line_4_5/1 -> d_id_line_4_5_block/2(State_iq_line_4_5_f0025), d_iq_line_4_5_block/2(State_iq_line_4_5_213cd), iq_bus_4_block/2(State_iq_line_4_5_86879), iq_bus_5_block/2(State_iq_line_4_5_0cb61)
  id_line_4_5/1 -> id_bus_4_block/2(State_id_line_4_5_a587b), d_id_line_4_5_block/1(State_id_line_4_5_42986), d_iq_line_4_5_block/1(State_id_line_4_5_3365c), id_bus_5_block/2(State_id_line_4_5_e8389)
  id_bus_6_block/1(Blockout_id_bus_6_c0a22) -> d_vd_bus_6_block/1(Alge_id_bus_6_7ffa8)
  id_bus_5_block/1(Blockout_id_bus_5_24227) -> d_vd_bus_5_block/1(Alge_id_bus_5_5b93e)
  id_bus_2_block/1(Blockout_id_bus_2_b293f) -> d_vd_bus_2_block/1(Alge_id_bus_2_c2beb)
  id_line_6_7/1 -> id_bus_6_block/3(State_id_line_6_7_daca9), d_id_line_6_7_block/1(State_id_line_6_7_bd89c), id_bus_7_block/2(State_id_line_6_7_c0e22), d_iq_line_6_7_block/1(State_id_line_6_7_f8f8d)
  iq_bus_4_block/1(Blockout_iq_bus_4_bba5d) -> d_vq_bus_4_block/1(Alge_iq_bus_4_34632)
  id_load_9/1 -> d_id_load_9_block/1(State_id_load_9_adb15), d_iq_load_9_block/1(State_id_load_9_c133f), id_bus_9_block/1(State_id_load_9_2a277)
  id_bus_4_block/1(Blockout_id_bus_4_81819) -> d_vd_bus_4_block/1(Alge_id_bus_4_4fdbe)
  vd_bus_1_out_block/1(Blockout_vd_bus_1_out_322ac) -> vd_bus_1_out/1
  vq_bus_1_out_block/1(Blockout_vq_bus_1_out_2811e) -> vq_bus_1_out/1
  iq_bus_3_block/1(Blockout_iq_bus_3_2e2f8) -> d_vq_bus_3_block/1(Alge_iq_bus_3_cccc7)
  vd_bus_6/1 -> d_vq_bus_6_block/2(State_vd_bus_6_2a50c), d_id_line_5_6_block/4(State_vd_bus_6_81e43), d_id_line_6_7_block/3(State_vd_bus_6_1b476), d_id_line_3_6_block/3(State_vd_bus_6_a863a)
  iq_bus_2_block/1(Blockout_iq_bus_2_7e5d3) -> d_vq_bus_2_block/1(Alge_iq_bus_2_afa01)
  vd_bus_2/1 -> vd_bus_2_out_block/1(State_vd_bus_2_cb137), d_vq_bus_2_block/2(State_vd_bus_2_6eee7), d_id_line_8_2_block/2(State_vd_bus_2_232dc)
  iq_line_6_7/1 -> d_iq_line_6_7_block/2(State_iq_line_6_7_dab1d), iq_bus_6_block/3(State_iq_line_6_7_26089), iq_bus_7_block/2(State_iq_line_6_7_e8477), d_id_line_6_7_block/2(State_iq_line_6_7_bf0cc)
  id_bus_1_block/1(Blockout_id_bus_1_1926f) -> d_vd_bus_1_block/1(Alge_id_bus_1_80866)
  iq_line_9_4/1 -> d_iq_line_9_4_block/2(State_iq_line_9_4_0d177), iq_bus_4_block/3(State_iq_line_9_4_6d8cb), iq_bus_9_block/3(State_iq_line_9_4_e3782), d_id_line_9_4_block/2(State_iq_line_9_4_6aab9)
  id_line_9_4/1 -> id_bus_4_block/3(State_id_line_9_4_59811), d_id_line_9_4_block/1(State_id_line_9_4_4873b), d_iq_line_9_4_block/1(State_id_line_9_4_42230), id_bus_9_block/3(State_id_line_9_4_cdab0)
  d_iq_line_8_9_block/1(Blockout_d_iq_line_8_9_1ac9c) -> iq_line_8_9/1
  d_iq_load_9_block/1(Blockout_d_iq_load_9_bcf8f) -> iq_load_9/1
  vd_bus_9/1 -> d_vq_bus_9_block/2(State_vd_bus_9_79c64), d_id_line_9_4_block/4(State_vd_bus_9_760c0), d_id_load_9_block/3(State_vd_bus_9_f7f95), d_id_line_8_9_block/4(State_vd_bus_9_4af5d)
  d_iq_line_7_8_block/1(Blockout_d_iq_line_7_8_0db81) -> iq_line_7_8/1
  vd_bus_2_out_block/1(Blockout_vd_bus_2_out_4b0bd) -> vd_bus_2_out/1
  d_vd_bus_9_block/1(Blockout_d_vd_bus_9_9824e) -> vd_bus_9/1
  d_vq_bus_9_block/1(Blockout_d_vq_bus_9_bd9e0) -> vq_bus_9/1
  iq_line_1_4/1 -> iq_bus_1_block/2(State_iq_line_1_4_ea68f), iq_bus_4_block/1(State_iq_line_1_4_ad230), d_id_line_1_4_block/1(State_iq_line_1_4_5b1cb)
  d_id_load_5_block/1(Blockout_d_id_load_5_45067) -> id_load_5/1
  vq_bus_7/1 -> d_vd_bus_7_block/2(State_vq_bus_7_85f46), d_iq_load_7_block/3(State_vq_bus_7_f7a5b), d_iq_line_6_7_block/4(State_vq_bus_7_7f00d), d_iq_line_7_8_block/3(State_vq_bus_7_6e292)
  d_vq_bus_3_block/1(Blockout_d_vq_bus_3_e2948) -> vq_bus_3/1
  iq_line_8_9/1 -> d_id_line_8_9_block/2(State_iq_line_8_9_a71ff), iq_bus_8_block/3(State_iq_line_8_9_dde8d), iq_bus_9_block/2(State_iq_line_8_9_a5789), d_iq_line_8_9_block/2(State_iq_line_8_9_3d23d)
  id_line_3_6/1 -> d_iq_line_3_6_block/1(State_id_line_3_6_009c9), id_bus_3_block/2(State_id_line_3_6_dffa3), id_bus_6_block/1(State_id_line_3_6_c2f24)
  id_line_8_9/1 -> id_bus_8_block/3(State_id_line_8_9_71460), d_id_line_8_9_block/1(State_id_line_8_9_588f7), d_iq_line_8_9_block/1(State_id_line_8_9_6201c), id_bus_9_block/2(State_id_line_8_9_39eb5)
  iq_line_7_8/1 -> d_id_line_7_8_block/2(State_iq_line_7_8_790f7), d_iq_line_7_8_block/2(State_iq_line_7_8_1b0e2), iq_bus_7_block/3(State_iq_line_7_8_380c1), iq_bus_8_block/1(State_iq_line_7_8_d1eb2)
  vd_bus_5/1 -> d_vq_bus_5_block/2(State_vd_bus_5_4af70), d_id_load_5_block/3(State_vd_bus_5_2ec2f), d_id_line_4_5_block/4(State_vd_bus_5_ce0e6), d_id_line_5_6_block/3(State_vd_bus_5_f7dd8)
  vd_bus_1/1 -> d_id_line_1_4_block/2(State_vd_bus_1_9b5a0), vd_bus_1_out_block/1(State_vd_bus_1_74d9b), d_vq_bus_1_block/2(State_vd_bus_1_380c1)
  iq_line_3_6/1 -> d_id_line_3_6_block/1(State_iq_line_3_6_057f5), iq_bus_3_block/2(State_iq_line_3_6_8c689), iq_bus_6_block/1(State_iq_line_3_6_b6d58)
  id_line_5_6/1 -> id_bus_6_block/2(State_id_line_5_6_c1efc), d_id_line_5_6_block/1(State_id_line_5_6_1a156), d_iq_line_5_6_block/1(State_id_line_5_6_c9e53), id_bus_5_block/3(State_id_line_5_6_04d6d)
  vq_bus_1/1 -> d_vd_bus_1_block/2(State_vq_bus_1_61947), d_iq_line_1_4_block/2(State_vq_bus_1_85cee), vq_bus_1_out_block/1(State_vq_bus_1_ae316)
  id_line_1_4/1 -> d_iq_line_1_4_block/1(State_id_line_1_4_423c5), id_bus_1_block/2(State_id_line_1_4_3f82b), id_bus_4_block/1(State_id_line_1_4_529f6)
  iq_load_9/1 -> d_id_load_9_block/2(State_iq_load_9_1d7e2), d_iq_load_9_block/2(State_iq_load_9_0ed41), iq_bus_9_block/1(State_iq_load_9_c7015)
  id_load_7/1 -> d_id_load_7_block/1(State_id_load_7_85756), id_bus_7_block/1(State_id_load_7_e82b6), d_iq_load_7_block/1(State_id_load_7_95f0d)
  iq_load_7/1 -> d_id_load_7_block/2(State_iq_load_7_0d377), d_iq_load_7_block/2(State_iq_load_7_fd2d1), iq_bus_7_block/1(State_iq_load_7_aef02)
  iq_load_5/1 -> d_id_load_5_block/2(State_iq_load_5_ef704), d_iq_load_5_block/2(State_iq_load_5_7c17a), iq_bus_5_block/1(State_iq_load_5_74a4d)
  vq_bus_8/1 -> d_vd_bus_8_block/2(State_vq_bus_8_ca02b), d_iq_line_8_2_block/3(State_vq_bus_8_09901), d_iq_line_7_8_block/4(State_vq_bus_8_9448a), d_iq_line_8_9_block/3(State_vq_bus_8_ba3ce)
  vd_bus_8/1 -> d_vq_bus_8_block/2(State_vd_bus_8_f2f43), d_id_line_8_2_block/3(State_vd_bus_8_a337d), d_id_line_8_9_block/3(State_vd_bus_8_8f873), d_id_line_7_8_block/4(State_vd_bus_8_e84a0)
  id_load_5/1 -> d_id_load_5_block/1(State_id_load_5_2b1bb), d_iq_load_5_block/1(State_id_load_5_10f5e), id_bus_5_block/1(State_id_load_5_f3160)
  vq_bus_9/1 -> d_vd_bus_9_block/2(State_vq_bus_9_fb0a9), d_iq_line_8_9_block/4(State_vq_bus_9_94e60), d_iq_load_9_block/3(State_vq_bus_9_4444e), d_iq_line_9_4_block/4(State_vq_bus_9_ed765)
  vd_bus_7/1 -> d_vq_bus_7_block/2(State_vd_bus_7_b9fb4), d_id_load_7_block/3(State_vd_bus_7_4e44c), d_id_line_6_7_block/4(State_vd_bus_7_39ba6), d_id_line_7_8_block/3(State_vd_bus_7_19431)
  vq_bus_6/1 -> d_vd_bus_6_block/2(State_vq_bus_6_8f435), d_iq_line_3_6_block/3(State_vq_bus_6_3dee8), d_iq_line_5_6_block/4(State_vq_bus_6_316f0), d_iq_line_6_7_block/3(State_vq_bus_6_46bfc)
  vq_bus_4/1 -> d_vd_bus_4_block/2(State_vq_bus_4_0d84f), d_iq_line_1_4_block/3(State_vq_bus_4_61231), d_iq_line_4_5_block/3(State_vq_bus_4_01a8c), d_iq_line_9_4_block/3(State_vq_bus_4_bde9c)
  vd_bus_3/1 -> d_vq_bus_3_block/2(State_vd_bus_3_d37be), d_id_line_3_6_block/2(State_vd_bus_3_1ec5f), vd_bus_3_out_block/1(State_vd_bus_3_ac381)
  vq_bus_3/1 -> d_iq_line_3_6_block/2(State_vq_bus_3_bedda), d_vd_bus_3_block/2(State_vq_bus_3_26672), vq_bus_3_out_block/1(State_vq_bus_3_e6988)
  d_vq_bus_5_block/1(Blockout_d_vq_bus_5_7aa33) -> vq_bus_5/1
  d_iq_line_1_4_block/1(Blockout_d_iq_line_1_4_8e08d) -> iq_line_1_4/1
  d_iq_line_3_6_block/1(Blockout_d_iq_line_3_6_efa2c) -> iq_line_3_6/1
  d_vd_bus_2_block/1(Blockout_d_vd_bus_2_9f603) -> vd_bus_2/1
  d_vd_bus_5_block/1(Blockout_d_vd_bus_5_d9166) -> vd_bus_5/1
  d_id_line_8_9_block/1(Blockout_d_id_line_8_9_1db1d) -> id_line_8_9/1
  d_id_line_5_6_block/1(Blockout_d_id_line_5_6_9f7f0) -> id_line_5_6/1
  d_iq_load_5_block/1(Blockout_d_iq_load_5_e7eeb) -> iq_load_5/1
  d_iq_line_5_6_block/1(Blockout_d_iq_line_5_6_dbe92) -> iq_line_5_6/1
  d_id_line_4_5_block/1(Blockout_d_id_line_4_5_192af) -> id_line_4_5/1
  d_id_line_7_8_block/1(Blockout_d_id_line_7_8_47088) -> id_line_7_8/1
  d_vq_bus_8_block/1(Blockout_d_vq_bus_8_bbe49) -> vq_bus_8/1
  d_id_load_9_block/1(Blockout_d_id_load_9_c2cf2) -> id_load_9/1
  d_iq_line_4_5_block/1(Blockout_d_iq_line_4_5_f1556) -> iq_line_4_5/1
  d_vq_bus_1_block/1(Blockout_d_vq_bus_1_1e70c) -> vq_bus_1/1
  d_vq_bus_6_block/1(Blockout_d_vq_bus_6_9f6d7) -> vq_bus_6/1
  d_vd_bus_7_block/1(Blockout_d_vd_bus_7_6d513) -> vd_bus_7/1
  d_iq_line_6_7_block/1(Blockout_d_iq_line_6_7_dacae) -> iq_line_6_7/1
  d_vd_bus_3_block/1(Blockout_d_vd_bus_3_85bef) -> vd_bus_3/1
  d_iq_line_9_4_block/1(Blockout_d_iq_line_9_4_c7246) -> iq_line_9_4/1
  d_iq_load_7_block/1(Blockout_d_iq_load_7_80412) -> iq_load_7/1
  d_vd_bus_6_block/1(Blockout_d_vd_bus_6_cbe78) -> vd_bus_6/1
  d_vd_bus_8_block/1(Blockout_d_vd_bus_8_71a28) -> vd_bus_8/1
  d_vq_bus_4_block/1(Blockout_d_vq_bus_4_1d44a) -> vq_bus_4/1
  d_vq_bus_7_block/1(Blockout_d_vq_bus_7_ac7ae) -> vq_bus_7/1

== system IEEE9_case/SG_D_1 ==
  v_d_SG_D_1 : Inport
  v_q_SG_D_1 : Inport  Port=2
  E_fd_SG_D_1 : Integrator  InitialCondition=1.9805513012329263
  Px_1_SG_D_1 : Integrator  InitialCondition=0.0
  Px_2_SG_D_1 : Integrator  InitialCondition=0.0
  Px_3_SG_D_1 : Integrator  InitialCondition=1.3587350977693559e-31
  R_f_SG_D_1 : Integrator  InitialCondition=13.371550642324015
  T_e_SG_D_1_block : Subsystem
  T_m_SG_D_1 : Integrator  InitialCondition=0.7201733550664303
  V_f_SG_D_1 : Integrator  InitialCondition=19.805513012329264
  d_E_fd_SG_D_1_block : Subsystem
  d_Px_1_SG_D_1_block : Subsystem
  d_Px_2_SG_D_1_block : Subsystem
  d_Px_3_SG_D_1_block : Subsystem
  d_R_f_SG_D_1_block : Subsystem
  d_T_m_SG_D_1_block : Subsystem
  d_V_f_SG_D_1_block : Subsystem
  d_psi_1d_SG_D_1_block : Subsystem
  d_psi_d_SG_D_1_block : Subsystem
  d_psi_fd_SG_D_1_block : Subsystem
  d_psi_gq_SG_D_1_block : Subsystem
  d_psi_kq_SG_D_1_block : Subsystem
  d_psi_q_SG_D_1_block : Subsystem
  d_theta_SG_D_1_block : Subsystem
  d_w_SG_D_1_block : Subsystem
  i_d_SG_D_1_block : Subsystem
  i_q_SG_D_1_block : Subsystem
  psi_1d_SG_D_1 : Integrator  InitialCondition=0.845823229911384
  psi_d_SG_D_1 : Integrator  InitialCondition=0.8151549036594502
  psi_fd_SG_D_1 : Integrator  InitialCondition=1.0003915942211292
  psi_gq_SG_D_1 : Integrator  InitialCondition=0.35728835356649113
  psi_kq_SG_D_1 : Integrator  InitialCondition=-0.5582630524476424
  psi_q_SG_D_1 : Integrator  InitialCondition=-0.580593574545548
  theta_SG_D_1 : Integrator  InitialCondition=0.6186381378069596
  theta_SG_D_1_out_block : Subsystem
  w_SG_D_1 : Integrator  InitialCondition=376.99111843077515
  w_SG_D_1_out_block : Subsystem
  i_d_SG_D_1 : Outport
  i_q_SG_D_1 : Outport  Port=2
  T_e_SG_D_1 : Outport  Port=3
  w_SG_D_1_out : Outport  Port=4
  theta_SG_D_1_out : Outport  Port=5
  wires:
  T_m_SG_D_1/1 -> d_T_m_SG_D_1_block/2(State_T_m_SG_D_1_3bd62), d_w_SG_D_1_block/2(State_T_m_SG_D_1_318e6)
  d_theta_SG_D_1_block/1(Blockout_d_theta_SG_D_1_678a9) -> theta_SG_D_1/1
  d_Px_1_SG_D_1_block/1(Blockout_d_Px_1_SG_D_1_5306e) -> Px_1_SG_D_1/1
  V_f_SG_D_1/1 -> d_E_fd_SG_D_1_block/2(State_V_f_SG_D_1_4d4c3), d_V_f_SG_D_1_block/14(State_V_f_SG_D_1_e7d4d)
  psi_kq_SG_D_1/1 -> d_psi_q_SG_D_1_block/2(State_psi_kq_SG_D_1_3d651), d_psi_gq_SG_D_1_block/3(State_psi_kq_SG_D_1_74a91), d_psi_gq_SG_D_1_block/5(State_psi_kq_SG_D_1_1d6bb), d_psi_kq_SG_D_1_block/4(State_psi_kq_SG_D_1_dfcd5), d_V_f_SG_D_1_block/10(State_psi_kq_SG_D_1_21f9c), d_w_SG_D_1_block/5(State_psi_kq_SG_D_1_b491e), i_d_SG_D_1_block/2(State_psi_kq_SG_D_1_f1a3f), d_psi_gq_SG_D_1_block/8(State_psi_kq_SG_D_1_5d42d), d_psi_kq_SG_D_1_block/2(State_psi_kq_SG_D_1_01b22), i_q_SG_D_1_block/2(State_psi_kq_SG_D_1_642ee), T_e_SG_D_1_block/3(State_psi_kq_SG_D_1_fce1a)
  w_SG_D_1_out_block/1(Blockout_w_SG_D_1_out_73f9d) -> w_SG_D_1_out/1
  w_SG_D_1/1 -> d_w_SG_D_1_block/1(State_w_SG_D_1_f1fc7), d_V_f_SG_D_1_block/13(State_w_SG_D_1_c12d0), d_psi_q_SG_D_1_block/9(State_w_SG_D_1_e9f82), d_psi_d_SG_D_1_block/9(State_w_SG_D_1_6f6c4), d_V_f_SG_D_1_block/8(State_w_SG_D_1_c628b), d_Px_1_SG_D_1_block/2(State_w_SG_D_1_bae23), d_Px_2_SG_D_1_block/4(State_w_SG_D_1_fb742), d_Px_3_SG_D_1_block/6(State_w_SG_D_1_3e7b9), d_theta_SG_D_1_block/1(State_w_SG_D_1_6c997), d_T_m_SG_D_1_block/1(State_w_SG_D_1_89d82), w_SG_D_1_out_block/1(State_w_SG_D_1_9aa86)
  d_T_m_SG_D_1_block/1(Blockout_d_T_m_SG_D_1_8e6e4) -> T_m_SG_D_1/1
  d_Px_2_SG_D_1_block/1(Blockout_d_Px_2_SG_D_1_88157) -> Px_2_SG_D_1/1
  d_Px_3_SG_D_1_block/1(Blockout_d_Px_3_SG_D_1_7e78e) -> Px_3_SG_D_1/1
  psi_q_SG_D_1/1 -> d_psi_d_SG_D_1_block/8(State_psi_q_SG_D_1_72117), d_psi_q_SG_D_1_block/3(State_psi_q_SG_D_1_a2647), d_psi_gq_SG_D_1_block/6(State_psi_q_SG_D_1_14317), d_psi_gq_SG_D_1_block/9(State_psi_q_SG_D_1_0f53e), d_psi_kq_SG_D_1_block/5(State_psi_q_SG_D_1_68fd5), d_w_SG_D_1_block/6(State_psi_q_SG_D_1_932f1), d_V_f_SG_D_1_block/7(State_psi_q_SG_D_1_46b84), i_d_SG_D_1_block/3(State_psi_q_SG_D_1_208f7), T_e_SG_D_1_block/4(State_psi_q_SG_D_1_125de), i_q_SG_D_1_block/3(State_psi_q_SG_D_1_76ae1), d_V_f_SG_D_1_block/11(State_psi_q_SG_D_1_e84eb), d_w_SG_D_1_block/7(State_psi_q_SG_D_1_cdd53), T_e_SG_D_1_block/5(State_psi_q_SG_D_1_d8f2c)
  psi_fd_SG_D_1/1 -> d_psi_fd_SG_D_1_block/2(State_psi_fd_SG_D_1_e725c), d_psi_fd_SG_D_1_block/4(State_psi_fd_SG_D_1_e1ea7), d_psi_fd_SG_D_1_block/7(State_psi_fd_SG_D_1_82032), d_psi_fd_SG_D_1_block/10(State_psi_fd_SG_D_1_8c18b), d_psi_d_SG_D_1_block/3(State_psi_fd_SG_D_1_3d49f), d_psi_1d_SG_D_1_block/5(State_psi_fd_SG_D_1_d1f9e), d_w_SG_D_1_block/10(State_psi_fd_SG_D_1_f25db), d_V_f_SG_D_1_block/6(State_psi_fd_SG_D_1_c395f), d_psi_1d_SG_D_1_block/2(State_psi_fd_SG_D_1_7c5ea), i_d_SG_D_1_block/7(State_psi_fd_SG_D_1_19090), i_q_SG_D_1_block/7(State_psi_fd_SG_D_1_7b602), T_e_SG_D_1_block/8(State_psi_fd_SG_D_1_a01cd)
  psi_gq_SG_D_1/1 -> d_psi_q_SG_D_1_block/1(State_psi_gq_SG_D_1_fe9b5), d_psi_gq_SG_D_1_block/1(State_psi_gq_SG_D_1_acc90), d_psi_gq_SG_D_1_block/2(State_psi_gq_SG_D_1_4b99c), d_psi_gq_SG_D_1_block/4(State_psi_gq_SG_D_1_13c6b), d_psi_gq_SG_D_1_block/7(State_psi_gq_SG_D_1_78c02), d_psi_kq_SG_D_1_block/1(State_psi_gq_SG_D_1_49d8b), d_psi_kq_SG_D_1_block/3(State_psi_gq_SG_D_1_47bd3), d_w_SG_D_1_block/4(State_psi_gq_SG_D_1_0a0d0), d_V_f_SG_D_1_block/9(State_psi_gq_SG_D_1_6c695), i_q_SG_D_1_block/1(State_psi_gq_SG_D_1_b3414), T_e_SG_D_1_block/2(State_psi_gq_SG_D_1_cded7), i_d_SG_D_1_block/1(State_psi_gq_SG_D_1_953b8)
  v_d_SG_D_1/1 -> d_psi_d_SG_D_1_block/4(Input_v_d_SG_D_1_42b00), d_psi_q_SG_D_1_block/4(Input_v_d_SG_D_1_aa1d3)
  v_q_SG_D_1/1 -> d_psi_d_SG_D_1_block/6(Input_v_q_SG_D_1_ee29c), d_psi_q_SG_D_1_block/6(Input_v_q_SG_D_1_6253c)
  theta_SG_D_1/1 -> d_psi_d_SG_D_1_block/5(State_theta_SG_D_1_3952e), i_d_SG_D_1_block/4(State_theta_SG_D_1_67276), d_psi_d_SG_D_1_block/7(State_theta_SG_D_1_113de), i_d_SG_D_1_block/8(State_theta_SG_D_1_fdfe6), i_q_SG_D_1_block/4(State_theta_SG_D_1_7319b), i_q_SG_D_1_block/8(State_theta_SG_D_1_dd7cd), d_psi_q_SG_D_1_block/5(State_theta_SG_D_1_e1395), d_psi_q_SG_D_1_block/7(State_theta_SG_D_1_1d708), theta_SG_D_1_out_block/1(State_theta_SG_D_1_a22d0)
  Px_1_SG_D_1/1 -> d_Px_2_SG_D_1_block/2(State_Px_1_SG_D_1_e7112), d_Px_2_SG_D_1_block/3(State_Px_1_SG_D_1_31a86), d_Px_3_SG_D_1_block/5(State_Px_1_SG_D_1_15fdf), d_Px_3_SG_D_1_block/4(State_Px_1_SG_D_1_a9a67), d_Px_1_SG_D_1_block/1(State_Px_1_SG_D_1_568ef)
  Px_2_SG_D_1/1 -> d_Px_2_SG_D_1_block/1(State_Px_2_SG_D_1_c858b), d_Px_3_SG_D_1_block/2(State_Px_2_SG_D_1_8d556), d_Px_3_SG_D_1_block/3(State_Px_2_SG_D_1_a6db1)
  d_E_fd_SG_D_1_block/1(Blockout_d_E_fd_SG_D_1_f9109) -> E_fd_SG_D_1/1
  psi_1d_SG_D_1/1 -> d_psi_fd_SG_D_1_block/3(State_psi_1d_SG_D_1_f54e2), d_psi_fd_SG_D_1_block/8(State_psi_1d_SG_D_1_10c91), d_psi_d_SG_D_1_block/1(State_psi_1d_SG_D_1_1f550), d_psi_1d_SG_D_1_block/1(State_psi_1d_SG_D_1_7d745), d_psi_1d_SG_D_1_block/3(State_psi_1d_SG_D_1_1205e), d_w_SG_D_1_block/8(State_psi_1d_SG_D_1_43d35), d_V_f_SG_D_1_block/4(State_psi_1d_SG_D_1_08cf6), i_d_SG_D_1_block/5(State_psi_1d_SG_D_1_26fc3), d_psi_fd_SG_D_1_block/5(State_psi_1d_SG_D_1_1f956), i_q_SG_D_1_block/5(State_psi_1d_SG_D_1_b02a1), T_e_SG_D_1_block/6(State_psi_1d_SG_D_1_22d02)
  psi_d_SG_D_1/1 -> d_psi_fd_SG_D_1_block/6(State_psi_d_SG_D_1_b0c4f), d_psi_fd_SG_D_1_block/9(State_psi_d_SG_D_1_cf887), d_psi_q_SG_D_1_block/8(State_psi_d_SG_D_1_0e471), d_psi_1d_SG_D_1_block/4(State_psi_d_SG_D_1_3c3e9), d_V_f_SG_D_1_block/12(State_psi_d_SG_D_1_cef7e), i_q_SG_D_1_block/6(State_psi_d_SG_D_1_d4abd), d_V_f_SG_D_1_block/5(State_psi_d_SG_D_1_540a1), T_e_SG_D_1_block/1(State_psi_d_SG_D_1_b48d8), d_w_SG_D_1_block/3(State_psi_d_SG_D_1_8ac56), d_psi_d_SG_D_1_block/2(State_psi_d_SG_D_1_ce2c6), i_d_SG_D_1_block/6(State_psi_d_SG_D_1_a79fb), T_e_SG_D_1_block/7(State_psi_d_SG_D_1_4849f), d_w_SG_D_1_block/9(State_psi_d_SG_D_1_a02c6)
  d_w_SG_D_1_block/1(Blockout_d_w_SG_D_1_3285d) -> w_SG_D_1/1
  d_V_f_SG_D_1_block/1(Blockout_d_V_f_SG_D_1_1691d) -> V_f_SG_D_1/1
  i_d_SG_D_1_block/1(Blockout_i_d_SG_D_1_09dc5) -> i_d_SG_D_1/1
  d_R_f_SG_D_1_block/1(Blockout_d_R_f_SG_D_1_506d3) -> R_f_SG_D_1/1
  d_psi_q_SG_D_1_block/1(Blockout_d_psi_q_SG_D_1_5ed42) -> psi_q_SG_D_1/1
  T_e_SG_D_1_block/1(Blockout_T_e_SG_D_1_44096) -> T_e_SG_D_1/1
  d_psi_d_SG_D_1_block/1(Blockout_d_psi_d_SG_D_1_736fa) -> psi_d_SG_D_1/1
  d_psi_kq_SG_D_1_block/1(Blockout_d_psi_kq_SG_D_1_c4f81) -> psi_kq_SG_D_1/1
  d_psi_gq_SG_D_1_block/1(Blockout_d_psi_gq_SG_D_1_5896d) -> psi_gq_SG_D_1/1
  theta_SG_D_1_out_block/1(Blockout_theta_SG_D_1_out_f2916) -> theta_SG_D_1_out/1
  d_psi_1d_SG_D_1_block/1(Blockout_d_psi_1d_SG_D_1_c59e9) -> psi_1d_SG_D_1/1
  i_q_SG_D_1_block/1(Blockout_i_q_SG_D_1_db7dd) -> i_q_SG_D_1/1
  R_f_SG_D_1/1 -> d_V_f_SG_D_1_block/2(State_R_f_SG_D_1_d66fb), d_R_f_SG_D_1_block/2(State_R_f_SG_D_1_1a98f)
  Px_3_SG_D_1/1 -> d_Px_3_SG_D_1_block/1(State_Px_3_SG_D_1_17088), d_V_f_SG_D_1_block/3(State_Px_3_SG_D_1_e7eea)
  E_fd_SG_D_1/1 -> d_V_f_SG_D_1_block/1(State_E_fd_SG_D_1_f8358), d_E_fd_SG_D_1_block/1(State_E_fd_SG_D_1_4ae7b), d_R_f_SG_D_1_block/1(State_E_fd_SG_D_1_74d9e), d_psi_fd_SG_D_1_block/1(State_E_fd_SG_D_1_aaf46)
  d_psi_fd_SG_D_1_block/1(Blockout_d_psi_fd_SG_D_1_0824e) -> psi_fd_SG_D_1/1
